simulink model "dynamics"  (R2023a)
settings: Solver=ode4  StartTime=0.0  StopTime=t_duration  FixedStep=dt  MaxStep=max_step_size  RelTol=relative_tolerance
undefined symbols (not defined in the file or in its folder): plant
settings Model: Creator=ndelurgio  LastModifiedBy=ndelurgio

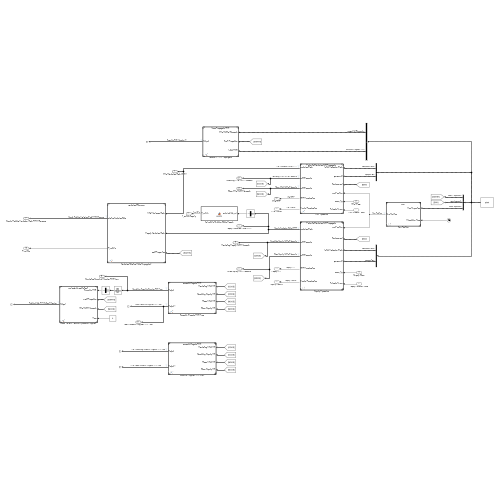
[thumbnail: Simulink's stored preview of the top-level diagram]
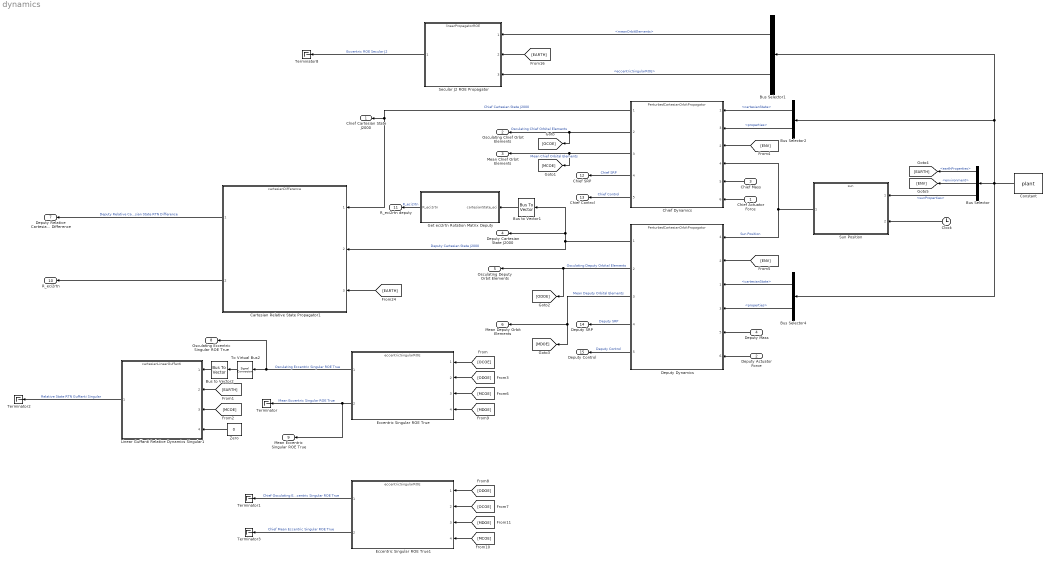
== system dynamics ==
  Chief Actuator Force : Inport  PortDimensions=3
  Deputy Actuator Force : Inport  Port=2  PortDimensions=3
  Chief Mass : Inport  Port=3
  Deputy Mass : Inport  Port=4
  Bus Selector : BusSelector  OutputSignals=environment.earthProperties,environment,environment.sunProperties
  Bus Selector1 : BusSelector  OutputSignals=chief.initialConditions.meanOrbitElements,deputy.initialConditions.eccentricSingularROE
  Bus Selector2 : BusSelector  OutputSignals=chief.initialConditions.cartesianState,chief.properties
  Bus Selector4 : BusSelector  OutputSignals=deputy.initialConditions.cartesianState,deputy.properties
  Bus to Vector1 : BusToVector
  Bus to Vector2 : BusToVector
  Cartesian Relative State Propagator1 : ModelReference  ModelNameDialog=cartesianDifference  SimulationMode=Normal  ModelReferenceVersion=1.35
  Chief Dynamics : ModelReference  ModelNameDialog=PerturbedCartesianOrbitPropagator.slx  SimulationMode=Normal  ModelReferenceVersion=1.163
      settings: PortSchema="{\"entries\":[{\"content\":{\"sides\":[{\"content\":{\"connectorIds\":[\"In1\",\"In3\",\"In2\",\"In4\",\"In5\",\"In6\"]},\"type\":\"ConnectorPlacement.EquallySpacedRectSide\",\"uuid\":\"0cdb5184-f322-4d12-8fb1-b7d6c888e918\"},{\"content\":{\"connectorIds\":[\"Out1\",\"Out2\",\"Out3\",\"Out4\",\"Out5\"],\"side\":\"RIGHT\"},\"type\":\"ConnectorPlacement.EquallySpacedRectSide\",\"uuid\":\"3b704699-bfdf-4090-ac04-9a1468a12d26\"},{\"content\":{\"side\":\"TOP\"},\"type\":\"ConnectorPlacement.EquallySpacedRectSide\",\"uuid\":\"efda26da-24ae-438b-9aa5-02661feb93c0\"}]},\"type\":\"ConnectorPlacement.EquallySpacedConnector\",\"uuid\":\"ad308b90-a5e4-431c-b4fb-02acb10c10ca\"}],\"packageUris\":[\"http://schema.mathworks.com/mf0/Connector/R2020b\"],\"version\":\"1.0\"}"
  Clock : Clock
  Constant : Constant  Value=plant  OutDataTypeStr=Bus: plantBus
  Deputy Dynamics : ModelReference  ModelNameDialog=PerturbedCartesianOrbitPropagator.slx  SimulationMode=Normal  ModelReferenceVersion=1.163
      settings: PortSchema="{\"entries\":[{\"content\":{\"sides\":[{\"content\":{\"connectorIds\":[\"In4\",\"In2\",\"In1\",\"In3\",\"In5\",\"In6\"]},\"type\":\"ConnectorPlacement.EquallySpacedRectSide\",\"uuid\":\"4c211678-740f-40f0-887b-605a3322d7cb\"},{\"content\":{\"connectorIds\":[\"Out1\",\"Out2\",\"Out3\",\"Out4\",\"Out5\"],\"side\":\"RIGHT\"},\"type\":\"ConnectorPlacement.EquallySpacedRectSide\",\"uuid\":\"7e8d6e44-a7a2-4633-9eac-45eb2a30ed1c\"},{\"content\":{\"side\":\"TOP\"},\"type\":\"ConnectorPlacement.EquallySpacedRectSide\",\"uuid\":\"00358f8f-509c-447f-b607-9e6e4b9aa7b5\"}]},\"type\":\"ConnectorPlacement.EquallySpacedConnector\",\"uuid\":\"f8258235-53bd-4241-8f5f-7f5c3c0a64eb\"}],\"packageUris\":[\"http://schema.mathworks.com/mf0/Connector/R2020b\"],\"version\":\"1.0\"}"
  Eccentric Singular ROE True : ModelReference  ModelNameDialog=eccentricSingularROE  SimulationMode=Normal  ModelReferenceVersion=1.13
  Eccentric Singular ROE True1 : ModelReference  ModelNameDialog=eccentricSingularROE  SimulationMode=Normal  ModelReferenceVersion=1.13
  Get eci2rtn Rotation Matrix Deputy : MATLAB Function  TreatAsAtomicUnit=on
  Linear Guffanti Relative Dynamics Singular1 : ModelReference  ModelNameDialog=cartesianLinearGuffanti  SimulationMode=Normal  ModelReferenceVersion=1.31
  Secular J2 ROE Propagator : ModelReference  ModelNameDialog=linearPropagatorROE  SimulationMode=Normal  ModelReferenceVersion=1.12
  Sun Position : ModelReference  ModelNameDialog=sun.slx  SimulationMode=Normal  ModelReferenceVersion=1.5
  Terminator{,1..3,8} (5 alike) : Terminator
  To Virtual Bus2 : SignalConversion  ConversionOutput=Virtual bus  OverrideOpt=off
  Zero : Constant  Value=0  OutDataTypeStr=Inherit: Inherit via back propagation
  Chief Cartesian State J2000 : Outport  OutDataTypeStr=Bus: cartesianState
  Osculating Chief Orbit Elements : Outport  Port=2  OutDataTypeStr=Bus: osculatingOrbitElements
  Mean Chief Orbit Elements : Outport  Port=3  OutDataTypeStr=Bus: meanOrbitElements
  Deputy Cartesian State J2000 : Outport  Port=4  OutDataTypeStr=Bus: cartesianState
  Osculating Deputy Orbit Elements : Outport  Port=5  OutDataTypeStr=Bus: osculatingOrbitElements
  Mean Deputy Orbit Elements : Outport  Port=6  OutDataTypeStr=Bus: meanOrbitElements
  Deputy Relative Cartesian State RTN Difference : Outport  Port=7  OutDataTypeStr=Bus: relativeCartesianState
  Osculating Eccentric Singular ROE True : Outport  Port=8  OutDataTypeStr=Bus: eccentricSingularROE
  Mean Eccentric Singular ROE True : Outport  Port=9  OutDataTypeStr=Bus: eccentricSingularROE
  R_eci2rtn : Outport  Port=10
  R_eci2rtn deputy : Outport  Port=11
  Chief SRP : Outport  Port=12
  Chief Control : Outport  Port=13  PortDimensions=3
  Deputy SRP : Outport  Port=14
  Deputy Control : Outport  Port=15  PortDimensions=3
  wires:
  Chief Dynamics/1 -> Chief Cartesian State J2000/1, Cartesian Relative State Propagator1/1  "Chief Cartesian State J2000"
  Eccentric Singular ROE True/1 -> Osculating Eccentric Singular ROE True/1, To Virtual Bus2/1  "Osculating Eccentric Singular ROE True"
  Secular J2 ROE Propagator/1 -> Terminator8/1  "Eccentric ROE Secular J2"
  Eccentric Singular ROE True/2 -> Terminator/1, Mean Eccentric Singular ROE True/1  "Mean Eccentric Singular ROE True"
  Chief Dynamics/2 -> [OCOE], Osculating Chief Orbit Elements/1  "Osculating Chief Orbital Elements"
  Chief Dynamics/3 -> [MCOE], Mean Chief Orbit Elements/1  "Mean Chief Orbital Elements"
  Deputy Dynamics/1 -> Cartesian Relative State Propagator1/2, Bus to Vector1/1, Deputy Cartesian State J2000/1  "Deputy Cartesian State J2000"
  Deputy Dynamics/2 -> [ODOE], Osculating Deputy Orbit Elements/1  "Osculating Deputy Orbital Elements"
  Deputy Dynamics/3 -> [MDOE], Mean Deputy Orbit Elements/1  "Mean Deputy Orbital Elements"
  [OCOE] -> Eccentric Singular ROE True/1
  [ODOE] -> Eccentric Singular ROE True/2
  [MCOE] -> Eccentric Singular ROE True/3
  [MDOE] -> Eccentric Singular ROE True/4
  Bus Selector1/2 -> Secular J2 ROE Propagator/3  "<eccentricSingularROE>"
  [EARTH] -> Secular J2 ROE Propagator/2
  Bus Selector1/1 -> Secular J2 ROE Propagator/1  "<meanOrbitElements>"
  Cartesian Relative State Propagator1/1 -> Deputy Relative Cartesian State RTN Difference/1  "Deputy Relative Cartesian State RTN Difference"
  [EARTH] -> Cartesian Relative State Propagator1/3
  [EARTH] -> Linear Guffanti Relative Dynamics Singular1/2
  [MCOE] -> Linear Guffanti Relative Dynamics Singular1/3
  Linear Guffanti Relative Dynamics Singular1/1 -> Terminator2/1  "Relative State RTN Guffanti Singular"
  Zero/1 -> Linear Guffanti Relative Dynamics Singular1/4
  Bus to Vector2/1 -> Linear Guffanti Relative Dynamics Singular1/1
  To Virtual Bus2/1 -> Bus to Vector2/1
  Bus Selector/3 -> Sun Position/1  "<sunProperties>"
  Clock/1 -> Sun Position/2
  Sun Position/1 -> Deputy Dynamics/4, Chief Dynamics/4  "Sun Position"
  Bus Selector/2 -> [ENV]  "<environment>"
  [ENV] -> Chief Dynamics/2
  [ENV] -> Deputy Dynamics/2
  Bus Selector2/1 -> Chief Dynamics/1  "<cartesianState>"
  Bus Selector2/2 -> Chief Dynamics/3  "<properties>"
  Constant/1 -> Bus Selector4/1, Bus Selector/1, Bus Selector1/1, Bus Selector2/1
  Bus Selector4/2 -> Deputy Dynamics/3  "<properties>"
  Bus Selector4/1 -> Deputy Dynamics/1  "<cartesianState>"
  Bus Selector/1 -> [EARTH]  "<earthProperties>"
  Chief Actuator Force/1 -> Chief Dynamics/6
  Deputy Actuator Force/1 -> Deputy Dynamics/6
  Chief Mass/1 -> Chief Dynamics/5
  Deputy Mass/1 -> Deputy Dynamics/5
  Cartesian Relative State Propagator1/2 -> R_eci2rtn/1
  [ODOE] -> Eccentric Singular ROE True1/1
  [MDOE] -> Eccentric Singular ROE True1/3
  [MCOE] -> Eccentric Singular ROE True1/4
  [OCOE] -> Eccentric Singular ROE True1/2
  Eccentric Singular ROE True1/2 -> Terminator3/1  "Chief Mean Eccentric Singular ROE True"
  Eccentric Singular ROE True1/1 -> Terminator1/1  "Chief Osculating Eccentric Singular ROE True"
  Bus to Vector1/1 -> Get eci2rtn Rotation Matrix Deputy/1(cartesianState_eci)
  Get eci2rtn Rotation Matrix Deputy/1(R_eci2rtn) -> R_eci2rtn deputy/1  "R_eci2rtn"
  Chief Dynamics/4 -> Chief SRP/1  "Chief SRP"
  Chief Dynamics/5 -> Chief Control/1  "Chief Control"
  Deputy Dynamics/5 -> Deputy Control/1  "Deputy Control"
  Deputy Dynamics/4 -> Deputy SRP/1  "Deputy SRP"

== matlab function dynamics/Get eci2rtn Rotation Matrix Deputy ==
  data: cartesianState_eci input; R_eci2rtn output
function R_eci2rtn  = eci2rtn(cartesianState_eci)

[~, R_eci2rtn] = eci2rtn(cartesianState_eci);

end
